simulink model "IIR_filter"  (R2017b)
settings: Solver=VariableStepAuto  StartTime=0.0  StopTime=10.0  RelTol=1e-3
libraries: dspstat3 x4, commutil2 x2, simulink x1
settings Model: Creator=ARNAB KUMAR MONDAL  LastModifiedBy=ARNAB KUMAR MONDAL

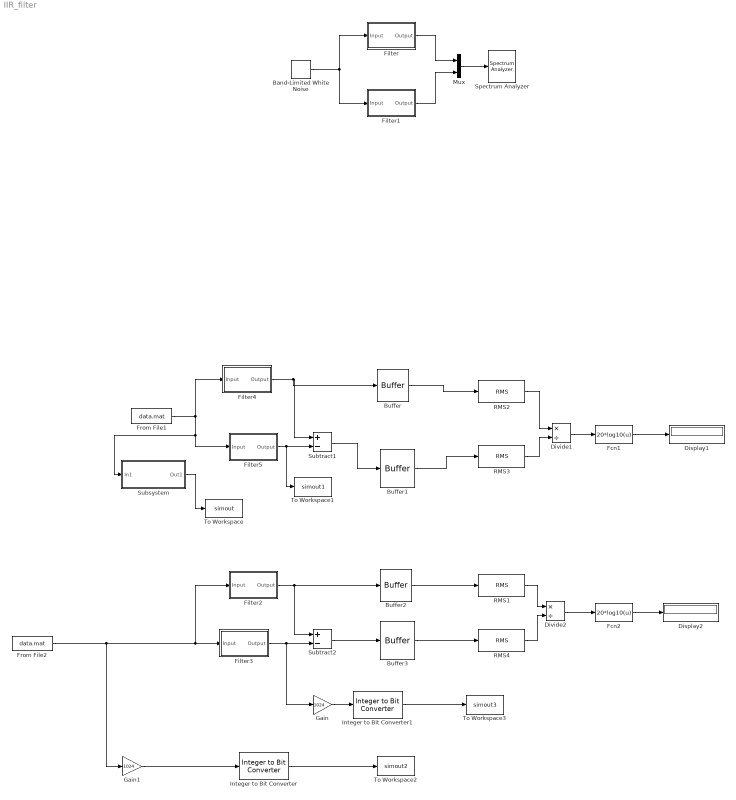
== system IIR_filter ==
  Band-Limited White Noise : simulink/Sources/Band-Limited White Noise  Cov=[1]  Ts=1/44100  seed=[23341]
  Buffer{,1..3} (4 alike) : Buffer  OutputFrames=off
  Display1 : Display
  Display2 : Display
  Divide1 : Product  Inputs=*/
  Divide2 : Product  Inputs=*/
  Fcn1 : Fcn  Expr=20*log10(u)
  Fcn2 : Fcn  Expr=20*log10(u)
  Filter : Subsystem  Tag=FilterWizardSubSystem
      settings: ErrorFcn=dspFilterRealizedInBasicElemsAlgLoopErrFcnCallback
  Filter1 : Subsystem  Tag=FilterWizardSubSystem  mask{k=11, s=4, ck=11}
      settings: ErrorFcn=dspFilterRealizedInBasicElemsAlgLoopErrFcnCallback
  Filter2 : Subsystem  Tag=FilterWizardSubSystem
      settings: ErrorFcn=dspFilterRealizedInBasicElemsAlgLoopErrFcnCallback
  Filter3 : Subsystem  Tag=FilterWizardSubSystem  mask{k=11, s=5, ck=11}
      settings: ErrorFcn=dspFilterRealizedInBasicElemsAlgLoopErrFcnCallback
  Filter4 : Subsystem  Tag=FilterWizardSubSystem
      settings: ErrorFcn=dspFilterRealizedInBasicElemsAlgLoopErrFcnCallback
  Filter5 : Subsystem  Tag=FilterWizardSubSystem  mask{k=8, s=4, ck=11}
      settings: ErrorFcn=dspFilterRealizedInBasicElemsAlgLoopErrFcnCallback
  From File1 : FromFile  FileName=data.mat  SampleTime=1/44100
  From File2 : FromFile  FileName=data.mat  SampleTime=1/44100
  Gain : Gain  Gain=1024
  Gain1 : Gain  Gain=1024
  Integer to Bit Converter : commutil2/Integer to Bit Converter  nbits=32  signedInputValues=Signed  bitOrder=MSB first  outDtype=Same as input
  Integer to Bit Converter1 : commutil2/Integer to Bit Converter  nbits=32  signedInputValues=Signed  bitOrder=MSB first  outDtype=Same as input
  Mux : Mux  Inputs=2
  RMS{1..4} (4 alike) : dspstat3/RMS  run=on  directionMode=Each column  dimension=1  reset_popup=None
  Spectrum Analyzer : SpectrumAnalyzer
  Subsystem : Subsystem  mask{k=8, s=4}
  Subtract1 : Sum  Inputs=+-
  Subtract2 : Sum  Inputs=+-
  To Workspace : ToWorkspace  VariableName=simout  SaveFormat=Timeseries  SampleTime=-1
  To Workspace1 : ToWorkspace  VariableName=simout1  SaveFormat=Timeseries  SampleTime=-1
  To Workspace2 : ToWorkspace  VariableName=simout2  SaveFormat=Timeseries  SampleTime=-1
      settings: Save2DSignal=2-D array (concatenate along first dimension)
  To Workspace3 : ToWorkspace  VariableName=simout3  SaveFormat=Timeseries  SampleTime=-1
      settings: Save2DSignal=2-D array (concatenate along first dimension)
  wires:
  Band-Limited White Noise/1 -> Filter/1(Input), Filter1/1(Input)
  Filter1/1(Output) -> Mux/2
  RMS2/1 -> Divide1/1
  Filter4/1(Output) -> Buffer/1, Subtract1/1
  Divide1/1 -> Fcn1/1
  From File1/1 -> Subsystem/1(In1), Filter5/1(Input), Filter4/1(Input)
  RMS3/1 -> Divide1/2
  Filter5/1(Output) -> To Workspace1/1, Subtract1/2
  Fcn1/1 -> Display1/1
  Subtract1/1 -> Buffer1/1
  Buffer/1 -> RMS2/1
  Buffer1/1 -> RMS3/1
  Fcn2/1 -> Display2/1
  Buffer3/1 -> RMS4/1
  Divide2/1 -> Fcn2/1
  RMS1/1 -> Divide2/1
  Subtract2/1 -> Buffer3/1
  Filter2/1(Output) -> Subtract2/1, Buffer2/1
  RMS4/1 -> Divide2/2
  Buffer2/1 -> RMS1/1
  Filter3/1(Output) -> Gain/1, Subtract2/2
  From File2/1 -> Filter2/1(Input), Filter3/1(Input), Gain1/1
  Subsystem/1(Out1) -> To Workspace/1
  Integer to Bit Converter/1 -> To Workspace2/1
  Integer to Bit Converter1/1 -> To Workspace3/1
  Gain1/1 -> Integer to Bit Converter/1
  Gain/1 -> Integer to Bit Converter1/1
  Filter/1(Output) -> Mux/1
  Mux/1 -> Spectrum Analyzer/1

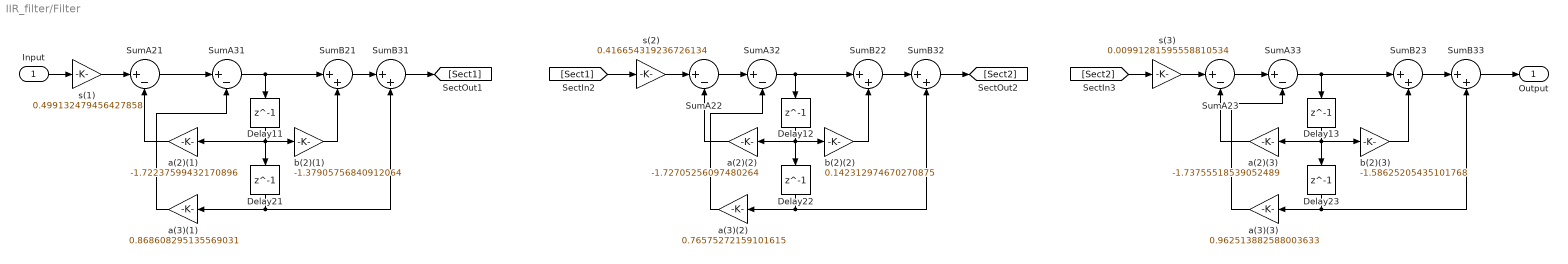
== system IIR_filter/Filter ==
  Input : Inport
  Delay{11..13,21..23} (6 alike) : Delay  DelayLength=1  InitialCondition=0
  SumA{21..23,31..33} (6 alike) : Sum  Inputs=|+-  RndMeth=Nearest  SaturateOnIntegerOverflow=on  OutDataTypeStr=Inherit: Same as first input
  SumB{21..23,31..33} (6 alike) : Sum  Inputs=|++  RndMeth=Nearest  SaturateOnIntegerOverflow=on  OutDataTypeStr=Inherit: Same as first input
  a(2)(1) : Gain  Gain=-1.72237599432170896  ParamDataTypeStr=double  RndMeth=Nearest  SaturateOnIntegerOverflow=on  OutDataTypeStr=Inherit: Same as input
  a(2)(2) : Gain  Gain=-1.72705256097480264  ParamDataTypeStr=double  RndMeth=Nearest  SaturateOnIntegerOverflow=on  OutDataTypeStr=Inherit: Same as input
  a(2)(3) : Gain  Gain=-1.73755518539052489  ParamDataTypeStr=double  RndMeth=Nearest  SaturateOnIntegerOverflow=on  OutDataTypeStr=Inherit: Same as input
  a(3)(1) : Gain  Gain=0.868608295135569031  ParamDataTypeStr=double  RndMeth=Nearest  SaturateOnIntegerOverflow=on  OutDataTypeStr=Inherit: Same as input
  a(3)(2) : Gain  Gain=0.76575272159101615  ParamDataTypeStr=double  RndMeth=Nearest  SaturateOnIntegerOverflow=on  OutDataTypeStr=Inherit: Same as input
  a(3)(3) : Gain  Gain=0.962513882588003633  ParamDataTypeStr=double  RndMeth=Nearest  SaturateOnIntegerOverflow=on  OutDataTypeStr=Inherit: Same as input
  b(2)(1) : Gain  Gain=-1.37905756840912064  ParamDataTypeStr=double  RndMeth=Nearest  SaturateOnIntegerOverflow=on  OutDataTypeStr=Inherit: Same as input
  b(2)(2) : Gain  Gain=0.142312974670270875  ParamDataTypeStr=double  RndMeth=Nearest  SaturateOnIntegerOverflow=on  OutDataTypeStr=Inherit: Same as input
  b(2)(3) : Gain  Gain=-1.58625205435101768  ParamDataTypeStr=double  RndMeth=Nearest  SaturateOnIntegerOverflow=on  OutDataTypeStr=Inherit: Same as input
  s(1) : Gain  Gain=0.499132479456427858  ParamDataTypeStr=double  RndMeth=Nearest  SaturateOnIntegerOverflow=on  OutDataTypeStr=Inherit: Same as input
  s(2) : Gain  Gain=0.416654319236726134  ParamDataTypeStr=double  RndMeth=Nearest  SaturateOnIntegerOverflow=on  OutDataTypeStr=Inherit: Same as input
  s(3) : Gain  Gain=0.00991281595558810534  ParamDataTypeStr=double  RndMeth=Nearest  SaturateOnIntegerOverflow=on  OutDataTypeStr=Inherit: Same as input
  Output : Outport
  wires:
  Input/1 -> s(1)/1
  s(1)/1 -> SumA21/1
  SumA21/1 -> SumA31/1
  SumA31/1 -> SumB21/1, Delay11/1
  SumB21/1 -> SumB31/1
  SumB31/1 -> [Sect1]
  a(2)(1)/1 -> SumA21/2
  Delay11/1 -> b(2)(1)/1, Delay21/1, a(2)(1)/1
  b(2)(1)/1 -> SumB21/2
  a(3)(1)/1 -> SumA31/2
  Delay21/1 -> SumB31/2, a(3)(1)/1
  [Sect1] -> s(2)/1
  s(2)/1 -> SumA22/1
  SumA22/1 -> SumA32/1
  SumA32/1 -> SumB22/1, Delay12/1
  SumB22/1 -> SumB32/1
  SumB32/1 -> [Sect2]
  a(2)(2)/1 -> SumA22/2
  Delay12/1 -> b(2)(2)/1, Delay22/1, a(2)(2)/1
  b(2)(2)/1 -> SumB22/2
  a(3)(2)/1 -> SumA32/2
  Delay22/1 -> SumB32/2, a(3)(2)/1
  b(2)(3)/1 -> SumB23/2
  SumA33/1 -> SumB23/1, Delay13/1
  [Sect2] -> s(3)/1
  Delay23/1 -> SumB33/2, a(3)(3)/1
  Delay13/1 -> b(2)(3)/1, Delay23/1, a(2)(3)/1
  SumB23/1 -> SumB33/1
  SumA23/1 -> SumA33/1
  a(3)(3)/1 -> SumA33/2
  s(3)/1 -> SumA23/1
  a(2)(3)/1 -> SumA23/2
  SumB33/1 -> Output/1

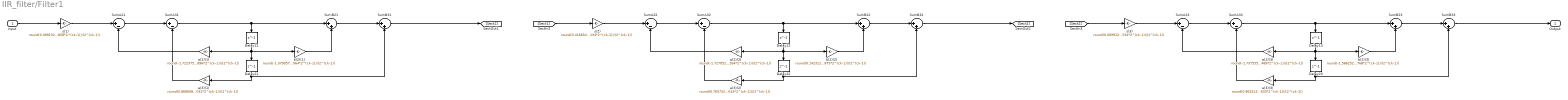
== system IIR_filter/Filter1 ==
  Input : Inport
  Delay{11..13,21..23} (6 alike) : Delay  DelayLength=1  InitialCondition=0
  SumA{21..23,31..33} (6 alike) : Sum  Inputs=|+-  RndMeth=Nearest  SaturateOnIntegerOverflow=on  OutDataTypeStr=Inherit: Same as first input
  SumB{21..23,31..33} (6 alike) : Sum  Inputs=|++  RndMeth=Nearest  SaturateOnIntegerOverflow=on  OutDataTypeStr=Inherit: Same as first input
  a(2)(1) : Gain  Gain=round(-1.72237599432170896*2^(ck-1))/(2^(ck-1))  ParamDataTypeStr=double  RndMeth=Nearest  SaturateOnIntegerOverflow=on  OutDataTypeStr=Inherit: Same as input
  a(2)(2) : Gain  Gain=round(-1.72705256097480264*2^(ck-1))/(2^(ck-1))  ParamDataTypeStr=double  RndMeth=Nearest  SaturateOnIntegerOverflow=on  OutDataTypeStr=Inherit: Same as input
  a(2)(3) : Gain  Gain=round(-1.73755518539052489*2^(ck-1))/(2^(ck-1))  ParamDataTypeStr=double  RndMeth=Nearest  SaturateOnIntegerOverflow=on  OutDataTypeStr=Inherit: Same as input
  a(3)(1) : Gain  Gain=round(0.868608295135569031*2^(ck-1))/(2^(ck-1))  ParamDataTypeStr=double  RndMeth=Nearest  SaturateOnIntegerOverflow=on  OutDataTypeStr=Inherit: Same as input
  a(3)(2) : Gain  Gain=round(0.76575272159101615*2^(ck-1))/(2^(ck-1))  ParamDataTypeStr=double  RndMeth=Nearest  SaturateOnIntegerOverflow=on  OutDataTypeStr=Inherit: Same as input
  a(3)(3) : Gain  Gain=round(0.962513882588003633*2^(ck-1))/(2^(ck-1))  ParamDataTypeStr=double  RndMeth=Nearest  SaturateOnIntegerOverflow=on  OutDataTypeStr=Inherit: Same as input
  b(2)(1) : Gain  Gain=round(-1.37905756840912064*2^(ck-1))/(2^(ck-1))  ParamDataTypeStr=double  RndMeth=Nearest  SaturateOnIntegerOverflow=on  OutDataTypeStr=Inherit: Same as input
  b(2)(2) : Gain  Gain=round(0.142312974670270875*2^(ck-1))/(2^(ck-1))  ParamDataTypeStr=double  RndMeth=Nearest  SaturateOnIntegerOverflow=on  OutDataTypeStr=Inherit: Same as input
  b(2)(3) : Gain  Gain=round(-1.58625205435101768*2^(ck-1))/(2^(ck-1))  ParamDataTypeStr=double  RndMeth=Nearest  SaturateOnIntegerOverflow=on  OutDataTypeStr=Inherit: Same as input
  s(1) : Gain  Gain=round(0.499132479456427858*2^(ck-1))/(2^(ck-1))  ParamDataTypeStr=double  RndMeth=Nearest  SaturateOnIntegerOverflow=on  OutDataTypeStr=Inherit: Same as input
  s(2) : Gain  Gain=round(0.416654319236726134*2^(ck-1))/(2^(ck-1))  ParamDataTypeStr=double  RndMeth=Nearest  SaturateOnIntegerOverflow=on  OutDataTypeStr=Inherit: Same as input
  s(3) : Gain  Gain=round(0.00991281595558810534*2^(ck-1))/(2^(ck-1))  ParamDataTypeStr=double  RndMeth=Nearest  SaturateOnIntegerOverflow=on  OutDataTypeStr=Inherit: Same as input
  Output : Outport
  wires:
  Input/1 -> s(1)/1
  s(1)/1 -> SumA21/1
  SumA21/1 -> SumA31/1
  SumA31/1 -> SumB21/1, Delay11/1
  SumB21/1 -> SumB31/1
  SumB31/1 -> [Sect1]
  a(2)(1)/1 -> SumA21/2
  Delay11/1 -> a(2)(1)/1, b(2)(1)/1, Delay21/1
  b(2)(1)/1 -> SumB21/2
  a(3)(1)/1 -> SumA31/2
  Delay21/1 -> a(3)(1)/1, SumB31/2
  [Sect1] -> s(2)/1
  s(2)/1 -> SumA22/1
  SumA22/1 -> SumA32/1
  SumA32/1 -> SumB22/1, Delay12/1
  SumB22/1 -> SumB32/1
  SumB32/1 -> [Sect2]
  a(2)(2)/1 -> SumA22/2
  Delay12/1 -> a(2)(2)/1, b(2)(2)/1, Delay22/1
  b(2)(2)/1 -> SumB22/2
  a(3)(2)/1 -> SumA32/2
  Delay22/1 -> a(3)(2)/1, SumB32/2
  [Sect2] -> s(3)/1
  s(3)/1 -> SumA23/1
  SumA23/1 -> SumA33/1
  SumA33/1 -> SumB23/1, Delay13/1
  SumB23/1 -> SumB33/1
  SumB33/1 -> Output/1
  a(2)(3)/1 -> SumA23/2
  Delay13/1 -> a(2)(3)/1, b(2)(3)/1, Delay23/1
  b(2)(3)/1 -> SumB23/2
  a(3)(3)/1 -> SumA33/2
  Delay23/1 -> a(3)(3)/1, SumB33/2

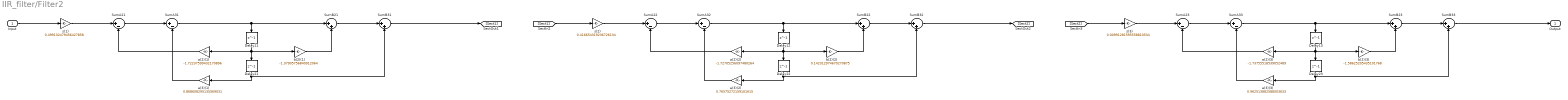
== system IIR_filter/Filter2 ==
  Input : Inport
  Delay{11..13,21..23} (6 alike) : Delay  DelayLength=1  InitialCondition=0
  SumA{21..23,31..33} (6 alike) : Sum  Inputs=|+-  RndMeth=Nearest  SaturateOnIntegerOverflow=on  OutDataTypeStr=Inherit: Same as first input
  SumB{21..23,31..33} (6 alike) : Sum  Inputs=|++  RndMeth=Nearest  SaturateOnIntegerOverflow=on  OutDataTypeStr=Inherit: Same as first input
  a(2)(1) : Gain  Gain=-1.72237599432170896  ParamDataTypeStr=double  RndMeth=Nearest  SaturateOnIntegerOverflow=on  OutDataTypeStr=Inherit: Same as input
  a(2)(2) : Gain  Gain=-1.72705256097480264  ParamDataTypeStr=double  RndMeth=Nearest  SaturateOnIntegerOverflow=on  OutDataTypeStr=Inherit: Same as input
  a(2)(3) : Gain  Gain=-1.73755518539052489  ParamDataTypeStr=double  RndMeth=Nearest  SaturateOnIntegerOverflow=on  OutDataTypeStr=Inherit: Same as input
  a(3)(1) : Gain  Gain=0.868608295135569031  ParamDataTypeStr=double  RndMeth=Nearest  SaturateOnIntegerOverflow=on  OutDataTypeStr=Inherit: Same as input
  a(3)(2) : Gain  Gain=0.76575272159101615  ParamDataTypeStr=double  RndMeth=Nearest  SaturateOnIntegerOverflow=on  OutDataTypeStr=Inherit: Same as input
  a(3)(3) : Gain  Gain=0.962513882588003633  ParamDataTypeStr=double  RndMeth=Nearest  SaturateOnIntegerOverflow=on  OutDataTypeStr=Inherit: Same as input
  b(2)(1) : Gain  Gain=-1.37905756840912064  ParamDataTypeStr=double  RndMeth=Nearest  SaturateOnIntegerOverflow=on  OutDataTypeStr=Inherit: Same as input
  b(2)(2) : Gain  Gain=0.142312974670270875  ParamDataTypeStr=double  RndMeth=Nearest  SaturateOnIntegerOverflow=on  OutDataTypeStr=Inherit: Same as input
  b(2)(3) : Gain  Gain=-1.58625205435101768  ParamDataTypeStr=double  RndMeth=Nearest  SaturateOnIntegerOverflow=on  OutDataTypeStr=Inherit: Same as input
  s(1) : Gain  Gain=0.499132479456427858  ParamDataTypeStr=double  RndMeth=Nearest  SaturateOnIntegerOverflow=on  OutDataTypeStr=Inherit: Same as input
  s(2) : Gain  Gain=0.416654319236726134  ParamDataTypeStr=double  RndMeth=Nearest  SaturateOnIntegerOverflow=on  OutDataTypeStr=Inherit: Same as input
  s(3) : Gain  Gain=0.00991281595558810534  ParamDataTypeStr=double  RndMeth=Nearest  SaturateOnIntegerOverflow=on  OutDataTypeStr=Inherit: Same as input
  Output : Outport
  wires:
  Input/1 -> s(1)/1
  s(1)/1 -> SumA21/1
  SumA21/1 -> SumA31/1
  SumA31/1 -> SumB21/1, Delay11/1
  SumB21/1 -> SumB31/1
  SumB31/1 -> [Sect1]
  a(2)(1)/1 -> SumA21/2
  Delay11/1 -> a(2)(1)/1, b(2)(1)/1, Delay21/1
  b(2)(1)/1 -> SumB21/2
  a(3)(1)/1 -> SumA31/2
  Delay21/1 -> a(3)(1)/1, SumB31/2
  [Sect1] -> s(2)/1
  s(2)/1 -> SumA22/1
  SumA22/1 -> SumA32/1
  SumA32/1 -> SumB22/1, Delay12/1
  SumB22/1 -> SumB32/1
  SumB32/1 -> [Sect2]
  a(2)(2)/1 -> SumA22/2
  Delay12/1 -> a(2)(2)/1, b(2)(2)/1, Delay22/1
  b(2)(2)/1 -> SumB22/2
  a(3)(2)/1 -> SumA32/2
  Delay22/1 -> a(3)(2)/1, SumB32/2
  [Sect2] -> s(3)/1
  s(3)/1 -> SumA23/1
  SumA23/1 -> SumA33/1
  SumA33/1 -> SumB23/1, Delay13/1
  SumB23/1 -> SumB33/1
  SumB33/1 -> Output/1
  a(2)(3)/1 -> SumA23/2
  Delay13/1 -> a(2)(3)/1, b(2)(3)/1, Delay23/1
  b(2)(3)/1 -> SumB23/2
  a(3)(3)/1 -> SumA33/2
  Delay23/1 -> a(3)(3)/1, SumB33/2

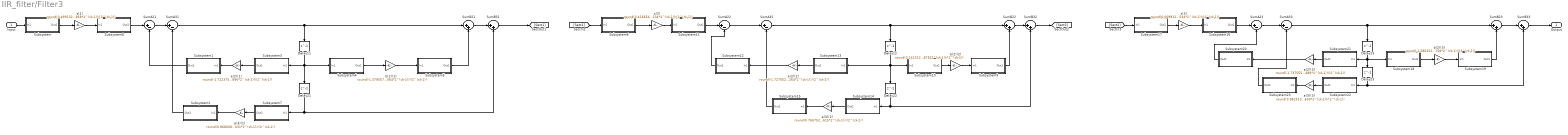
== system IIR_filter/Filter3 ==
  Input : Inport
  Delay{11..13,21..23} (6 alike) : Delay  DelayLength=1  InitialCondition=0
  Subsystem : Subsystem
  Subsystem1 : Subsystem
  Subsystem10 : Subsystem
  Subsystem11 : Subsystem
  Subsystem12 : Subsystem
  Subsystem13 : Subsystem
  Subsystem14 : Subsystem
  Subsystem15 : Subsystem
  Subsystem16 : Subsystem
  Subsystem17 : Subsystem
  Subsystem18 : Subsystem
  Subsystem19 : Subsystem
  Subsystem2 : Subsystem
  Subsystem20 : Subsystem
  Subsystem21 : Subsystem
  Subsystem22 : Subsystem
  Subsystem23 : Subsystem
  Subsystem3 : Subsystem
  Subsystem4 : Subsystem
  Subsystem5 : Subsystem
  Subsystem6 : Subsystem
  Subsystem7 : Subsystem
  Subsystem8 : Subsystem
  Subsystem9 : Subsystem
  SumA{21..23,31..33} (6 alike) : Sum  Inputs=|+-  RndMeth=Nearest  SaturateOnIntegerOverflow=on  OutDataTypeStr=Inherit: Same as first input
  SumB{21..23,31..33} (6 alike) : Sum  Inputs=|++  RndMeth=Nearest  SaturateOnIntegerOverflow=on  OutDataTypeStr=Inherit: Same as first input
  a(2)(1) : Gain  Gain=round(-1.72237599432170896*2^(ck-1))/(2^(ck-1))  ParamDataTypeStr=double  RndMeth=Nearest  SaturateOnIntegerOverflow=on  OutDataTypeStr=Inherit: Same as input
  a(2)(2) : Gain  Gain=round(-1.72705256097480264*2^(ck-1))/(2^(ck-1))  ParamDataTypeStr=double  RndMeth=Nearest  SaturateOnIntegerOverflow=on  OutDataTypeStr=Inherit: Same as input
  a(2)(3) : Gain  Gain=round(-1.73755518539052489*2^(ck-1))/(2^(ck-1))  ParamDataTypeStr=double  RndMeth=Nearest  SaturateOnIntegerOverflow=on  OutDataTypeStr=Inherit: Same as input
  a(3)(1) : Gain  Gain=round(0.868608295135569031*2^(ck-1))/(2^(ck-1))  ParamDataTypeStr=double  RndMeth=Nearest  SaturateOnIntegerOverflow=on  OutDataTypeStr=Inherit: Same as input
  a(3)(2) : Gain  Gain=round(0.76575272159101615*2^(ck-1))/(2^(ck-1))  ParamDataTypeStr=double  RndMeth=Nearest  SaturateOnIntegerOverflow=on  OutDataTypeStr=Inherit: Same as input
  a(3)(3) : Gain  Gain=round(0.962513882588003633*2^(ck-1))/(2^(ck-1))  ParamDataTypeStr=double  RndMeth=Nearest  SaturateOnIntegerOverflow=on  OutDataTypeStr=Inherit: Same as input
  b(2)(1) : Gain  Gain=round(-1.37905756840912064*2^(ck-1))/(2^(ck-1))  ParamDataTypeStr=double  RndMeth=Nearest  SaturateOnIntegerOverflow=on  OutDataTypeStr=Inherit: Same as input
  b(2)(2) : Gain  Gain=round(0.142312974670270875*2^(ck-1))/(2^(ck-1))  ParamDataTypeStr=double  RndMeth=Nearest  SaturateOnIntegerOverflow=on  OutDataTypeStr=Inherit: Same as input
  b(2)(3) : Gain  Gain=round(-1.58625205435101768*2^(ck-1))/(2^(ck-1))  ParamDataTypeStr=double  RndMeth=Nearest  SaturateOnIntegerOverflow=on  OutDataTypeStr=Inherit: Same as input
  s(1) : Gain  Gain=round(0.499132479456427858*2^(ck-1))/(2^(ck-1))  ParamDataTypeStr=double  RndMeth=Nearest  SaturateOnIntegerOverflow=on  OutDataTypeStr=Inherit: Same as input
  s(2) : Gain  Gain=round(0.416654319236726134*2^(ck-1))/(2^(ck-1))  ParamDataTypeStr=double  RndMeth=Nearest  SaturateOnIntegerOverflow=on  OutDataTypeStr=Inherit: Same as input
  s(3) : Gain  Gain=round(0.00991281595558810534*2^(ck-1))/(2^(ck-1))  ParamDataTypeStr=double  RndMeth=Nearest  SaturateOnIntegerOverflow=on  OutDataTypeStr=Inherit: Same as input
  Output : Outport
  wires:
  SumB31/1 -> [Sect1]
  Delay11/1 -> Delay21/1, Subsystem4/1(In1), Subsystem3/1(In1)
  b(2)(1)/1 -> Subsystem5/1(In1)
  a(3)(1)/1 -> Subsystem2/1(In1)
  [Sect1] -> Subsystem6/1(In1)
  s(2)/1 -> Subsystem11/1(In1)
  SumB32/1 -> [Sect2]
  a(2)(2)/1 -> Subsystem12/1(In1)
  Delay12/1 -> Subsystem10/1(In1), Delay22/1, Subsystem13/1(In1)
  b(2)(2)/1 -> Subsystem9/1(In1)
  a(3)(2)/1 -> Subsystem15/1(In1)
  [Sect2] -> Subsystem17/1(In1)
  s(3)/1 -> Subsystem16/1(In1)
  a(2)(3)/1 -> Subsystem20/1(In1)
  Delay13/1 -> Subsystem21/1(In1), Delay23/1, Subsystem18/1(In1)
  b(2)(3)/1 -> Subsystem19/1(In1)
  a(3)(3)/1 -> Subsystem23/1(In1)
  s(1)/1 -> Subsystem8/1(In1)
  a(2)(1)/1 -> Subsystem1/1(In1)
  Input/1 -> Subsystem/1(In1)
  Subsystem/1(Out1) -> s(1)/1
  Subsystem1/1(Out1) -> SumA21/2
  Subsystem2/1(Out1) -> SumA31/2
  Subsystem3/1(Out1) -> a(2)(1)/1
  Subsystem4/1(Out1) -> b(2)(1)/1
  Subsystem5/1(Out1) -> SumB21/2
  Subsystem6/1(Out1) -> s(2)/1
  Subsystem7/1(Out1) -> a(3)(1)/1
  Subsystem8/1(Out1) -> SumA21/1
  Subsystem9/1(Out1) -> SumB22/2
  Subsystem10/1(Out1) -> b(2)(2)/1
  Subsystem11/1(Out1) -> SumA22/1
  Subsystem13/1(Out1) -> a(2)(2)/1
  Subsystem14/1(Out1) -> a(3)(2)/1
  Subsystem12/1(Out1) -> SumA22/2
  Subsystem15/1(Out1) -> SumA32/2
  Subsystem17/1(Out1) -> s(3)/1
  Subsystem19/1(Out1) -> SumB23/2
  Subsystem18/1(Out1) -> b(2)(3)/1
  Subsystem20/1(Out1) -> SumA23/2
  Subsystem21/1(Out1) -> a(2)(3)/1
  Subsystem22/1(Out1) -> a(3)(3)/1
  Subsystem23/1(Out1) -> SumA33/2
  Subsystem16/1(Out1) -> SumA23/1
  Delay21/1 -> SumB31/2, Subsystem7/1(In1)
  Delay22/1 -> SumB32/2, Subsystem14/1(In1)
  Delay23/1 -> SumB33/2, Subsystem22/1(In1)
  SumA21/1 -> SumA31/1
  SumB21/1 -> SumB31/1
  SumA22/1 -> SumA32/1
  SumB22/1 -> SumB32/1
  SumA23/1 -> SumA33/1
  SumB23/1 -> SumB33/1
  SumB33/1 -> Output/1
  SumA33/1 -> SumB23/1, Delay13/1
  SumA32/1 -> SumB22/1, Delay12/1
  SumA31/1 -> SumB21/1, Delay11/1

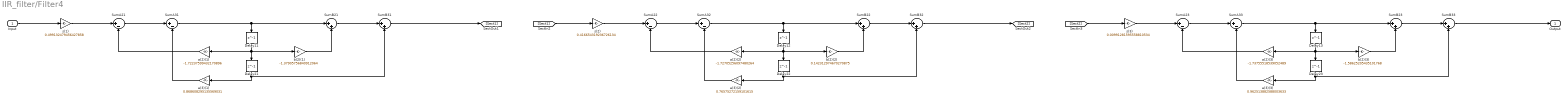
== system IIR_filter/Filter4 ==
  Input : Inport
  Delay{11..13,21..23} (6 alike) : Delay  DelayLength=1  InitialCondition=0
  SumA{21..23,31..33} (6 alike) : Sum  Inputs=|+-  RndMeth=Nearest  SaturateOnIntegerOverflow=on  OutDataTypeStr=Inherit: Same as first input
  SumB{21..23,31..33} (6 alike) : Sum  Inputs=|++  RndMeth=Nearest  SaturateOnIntegerOverflow=on  OutDataTypeStr=Inherit: Same as first input
  a(2)(1) : Gain  Gain=-1.72237599432170896  ParamDataTypeStr=double  RndMeth=Nearest  SaturateOnIntegerOverflow=on  OutDataTypeStr=Inherit: Same as input
  a(2)(2) : Gain  Gain=-1.72705256097480264  ParamDataTypeStr=double  RndMeth=Nearest  SaturateOnIntegerOverflow=on  OutDataTypeStr=Inherit: Same as input
  a(2)(3) : Gain  Gain=-1.73755518539052489  ParamDataTypeStr=double  RndMeth=Nearest  SaturateOnIntegerOverflow=on  OutDataTypeStr=Inherit: Same as input
  a(3)(1) : Gain  Gain=0.868608295135569031  ParamDataTypeStr=double  RndMeth=Nearest  SaturateOnIntegerOverflow=on  OutDataTypeStr=Inherit: Same as input
  a(3)(2) : Gain  Gain=0.76575272159101615  ParamDataTypeStr=double  RndMeth=Nearest  SaturateOnIntegerOverflow=on  OutDataTypeStr=Inherit: Same as input
  a(3)(3) : Gain  Gain=0.962513882588003633  ParamDataTypeStr=double  RndMeth=Nearest  SaturateOnIntegerOverflow=on  OutDataTypeStr=Inherit: Same as input
  b(2)(1) : Gain  Gain=-1.37905756840912064  ParamDataTypeStr=double  RndMeth=Nearest  SaturateOnIntegerOverflow=on  OutDataTypeStr=Inherit: Same as input
  b(2)(2) : Gain  Gain=0.142312974670270875  ParamDataTypeStr=double  RndMeth=Nearest  SaturateOnIntegerOverflow=on  OutDataTypeStr=Inherit: Same as input
  b(2)(3) : Gain  Gain=-1.58625205435101768  ParamDataTypeStr=double  RndMeth=Nearest  SaturateOnIntegerOverflow=on  OutDataTypeStr=Inherit: Same as input
  s(1) : Gain  Gain=0.499132479456427858  ParamDataTypeStr=double  RndMeth=Nearest  SaturateOnIntegerOverflow=on  OutDataTypeStr=Inherit: Same as input
  s(2) : Gain  Gain=0.416654319236726134  ParamDataTypeStr=double  RndMeth=Nearest  SaturateOnIntegerOverflow=on  OutDataTypeStr=Inherit: Same as input
  s(3) : Gain  Gain=0.00991281595558810534  ParamDataTypeStr=double  RndMeth=Nearest  SaturateOnIntegerOverflow=on  OutDataTypeStr=Inherit: Same as input
  Output : Outport
  wires:
  Input/1 -> s(1)/1
  s(1)/1 -> SumA21/1
  SumA21/1 -> SumA31/1
  SumA31/1 -> SumB21/1, Delay11/1
  SumB21/1 -> SumB31/1
  SumB31/1 -> [Sect1]
  a(2)(1)/1 -> SumA21/2
  Delay11/1 -> a(2)(1)/1, b(2)(1)/1, Delay21/1
  b(2)(1)/1 -> SumB21/2
  a(3)(1)/1 -> SumA31/2
  Delay21/1 -> a(3)(1)/1, SumB31/2
  [Sect1] -> s(2)/1
  s(2)/1 -> SumA22/1
  SumA22/1 -> SumA32/1
  SumA32/1 -> SumB22/1, Delay12/1
  SumB22/1 -> SumB32/1
  SumB32/1 -> [Sect2]
  a(2)(2)/1 -> SumA22/2
  Delay12/1 -> a(2)(2)/1, b(2)(2)/1, Delay22/1
  b(2)(2)/1 -> SumB22/2
  a(3)(2)/1 -> SumA32/2
  Delay22/1 -> a(3)(2)/1, SumB32/2
  [Sect2] -> s(3)/1
  s(3)/1 -> SumA23/1
  SumA23/1 -> SumA33/1
  SumA33/1 -> SumB23/1, Delay13/1
  SumB23/1 -> SumB33/1
  SumB33/1 -> Output/1
  a(2)(3)/1 -> SumA23/2
  Delay13/1 -> a(2)(3)/1, b(2)(3)/1, Delay23/1
  b(2)(3)/1 -> SumB23/2
  a(3)(3)/1 -> SumA33/2
  Delay23/1 -> a(3)(3)/1, SumB33/2

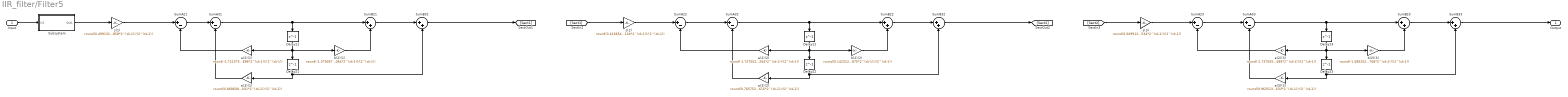
== system IIR_filter/Filter5 ==
  Input : Inport
  Delay{11..13,21..23} (6 alike) : Delay  DelayLength=1  InitialCondition=0
  Subsystem : Subsystem
  SumA{21..23,31..33} (6 alike) : Sum  Inputs=|+-  RndMeth=Nearest  SaturateOnIntegerOverflow=on  OutDataTypeStr=Inherit: Same as first input
  SumB{21..23,31..33} (6 alike) : Sum  Inputs=|++  RndMeth=Nearest  SaturateOnIntegerOverflow=on  OutDataTypeStr=Inherit: Same as first input
  a(2)(1) : Gain  Gain=round(-1.72237599432170896*2^(ck-1))/(2^(ck-1))  ParamDataTypeStr=double  RndMeth=Nearest  SaturateOnIntegerOverflow=on  OutDataTypeStr=Inherit: Same as input
  a(2)(2) : Gain  Gain=round(-1.72705256097480264*2^(ck-1))/(2^(ck-1))  ParamDataTypeStr=double  RndMeth=Nearest  SaturateOnIntegerOverflow=on  OutDataTypeStr=Inherit: Same as input
  a(2)(3) : Gain  Gain=round(-1.73755518539052489*2^(ck-1))/(2^(ck-1))  ParamDataTypeStr=double  RndMeth=Nearest  SaturateOnIntegerOverflow=on  OutDataTypeStr=Inherit: Same as input
  a(3)(1) : Gain  Gain=round(0.868608295135569031*2^(ck-1))/(2^(ck-1))  ParamDataTypeStr=double  RndMeth=Nearest  SaturateOnIntegerOverflow=on  OutDataTypeStr=Inherit: Same as input
  a(3)(2) : Gain  Gain=round(0.76575272159101615*2^(ck-1))/(2^(ck-1))  ParamDataTypeStr=double  RndMeth=Nearest  SaturateOnIntegerOverflow=on  OutDataTypeStr=Inherit: Same as input
  a(3)(3) : Gain  Gain=round(0.962513882588003633*2^(ck-1))/(2^(ck-1))  ParamDataTypeStr=double  RndMeth=Nearest  SaturateOnIntegerOverflow=on  OutDataTypeStr=Inherit: Same as input
  b(2)(1) : Gain  Gain=round(-1.37905756840912064*2^(ck-1))/(2^(ck-1))  ParamDataTypeStr=double  RndMeth=Nearest  SaturateOnIntegerOverflow=on  OutDataTypeStr=Inherit: Same as input
  b(2)(2) : Gain  Gain=round(0.142312974670270875*2^(ck-1))/(2^(ck-1))  ParamDataTypeStr=double  RndMeth=Nearest  SaturateOnIntegerOverflow=on  OutDataTypeStr=Inherit: Same as input
  b(2)(3) : Gain  Gain=round(-1.58625205435101768*2^(ck-1))/(2^(ck-1))  ParamDataTypeStr=double  RndMeth=Nearest  SaturateOnIntegerOverflow=on  OutDataTypeStr=Inherit: Same as input
  s(1) : Gain  Gain=round(0.499132479456427858*2^(ck-1))/(2^(ck-1))  ParamDataTypeStr=double  RndMeth=Nearest  SaturateOnIntegerOverflow=on  OutDataTypeStr=Inherit: Same as input
  s(2) : Gain  Gain=round(0.416654319236726134*2^(ck-1))/(2^(ck-1))  ParamDataTypeStr=double  RndMeth=Nearest  SaturateOnIntegerOverflow=on  OutDataTypeStr=Inherit: Same as input
  s(3) : Gain  Gain=round(0.00991281595558810534*2^(ck-1))/(2^(ck-1))  ParamDataTypeStr=double  RndMeth=Nearest  SaturateOnIntegerOverflow=on  OutDataTypeStr=Inherit: Same as input
  Output : Outport
  wires:
  SumB21/1 -> SumB31/1
  SumB31/1 -> [Sect1]
  Delay11/1 -> a(2)(1)/1, b(2)(1)/1, Delay21/1
  b(2)(1)/1 -> SumB21/2
  a(3)(1)/1 -> SumA31/2
  Delay21/1 -> a(3)(1)/1, SumB31/2
  [Sect1] -> s(2)/1
  s(2)/1 -> SumA22/1
  SumA22/1 -> SumA32/1
  SumA32/1 -> SumB22/1, Delay12/1
  SumB22/1 -> SumB32/1
  SumB32/1 -> [Sect2]
  a(2)(2)/1 -> SumA22/2
  Delay12/1 -> a(2)(2)/1, b(2)(2)/1, Delay22/1
  b(2)(2)/1 -> SumB22/2
  a(3)(2)/1 -> SumA32/2
  Delay22/1 -> a(3)(2)/1, SumB32/2
  [Sect2] -> s(3)/1
  s(3)/1 -> SumA23/1
  SumA23/1 -> SumA33/1
  SumA33/1 -> SumB23/1, Delay13/1
  SumB23/1 -> SumB33/1
  a(2)(3)/1 -> SumA23/2
  Delay13/1 -> a(2)(3)/1, b(2)(3)/1, Delay23/1
  b(2)(3)/1 -> SumB23/2
  a(3)(3)/1 -> SumA33/2
  Delay23/1 -> a(3)(3)/1, SumB33/2
  s(1)/1 -> SumA21/1
  SumA21/1 -> SumA31/1
  a(2)(1)/1 -> SumA21/2
  SumA31/1 -> SumB21/1, Delay11/1
  Input/1 -> Subsystem/1(In1)
  Subsystem/1(Out1) -> s(1)/1
  SumB33/1 -> Output/1

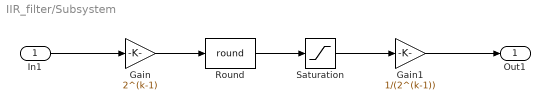
== system IIR_filter/Subsystem ==
  In1 : Inport
  Gain : Gain  Gain=2^(k-1)
  Gain1 : Gain  Gain=1/(2^(k-1))
  Round : Rounding  Operator=round
  Saturation : Saturate  UpperLimit=2^(k+s+-1)-1  LowerLimit=-2^(k+s-1)
  Out1 : Outport
  wires:
  Round/1 -> Saturation/1
  Saturation/1 -> Gain1/1
  Gain/1 -> Round/1
  In1/1 -> Gain/1
  Gain1/1 -> Out1/1

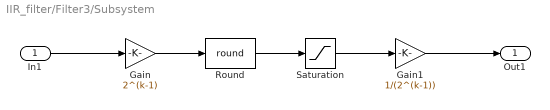
== system IIR_filter/Filter3/Subsystem ==
  In1 : Inport
  Gain : Gain  Gain=2^(k-1)
  Gain1 : Gain  Gain=1/(2^(k-1))
  Round : Rounding  Operator=round
  Saturation : Saturate  UpperLimit=2^(k+s+-1)-1  LowerLimit=-2^(k+s-1)
  Out1 : Outport
  wires:
  Round/1 -> Saturation/1
  Saturation/1 -> Gain1/1
  Gain/1 -> Round/1
  In1/1 -> Gain/1
  Gain1/1 -> Out1/1

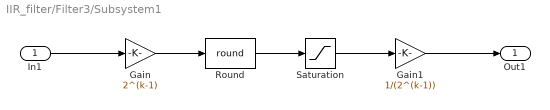
== system IIR_filter/Filter3/Subsystem1 ==
  In1 : Inport
  Gain : Gain  Gain=2^(k-1)
  Gain1 : Gain  Gain=1/(2^(k-1))
  Round : Rounding  Operator=round
  Saturation : Saturate  UpperLimit=2^(k+s+-1)-1  LowerLimit=-2^(k+s-1)
  Out1 : Outport
  wires:
  Round/1 -> Saturation/1
  Saturation/1 -> Gain1/1
  Gain/1 -> Round/1
  In1/1 -> Gain/1
  Gain1/1 -> Out1/1

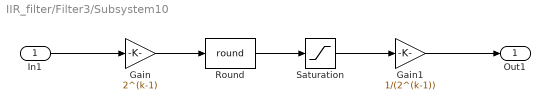
== system IIR_filter/Filter3/Subsystem10 ==
  In1 : Inport
  Gain : Gain  Gain=2^(k-1)
  Gain1 : Gain  Gain=1/(2^(k-1))
  Round : Rounding  Operator=round
  Saturation : Saturate  UpperLimit=2^(k+s+-1)-1  LowerLimit=-2^(k+s-1)
  Out1 : Outport
  wires:
  Round/1 -> Saturation/1
  Saturation/1 -> Gain1/1
  Gain/1 -> Round/1
  In1/1 -> Gain/1
  Gain1/1 -> Out1/1

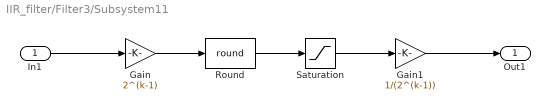
== system IIR_filter/Filter3/Subsystem11 ==
  In1 : Inport
  Gain : Gain  Gain=2^(k-1)
  Gain1 : Gain  Gain=1/(2^(k-1))
  Round : Rounding  Operator=round
  Saturation : Saturate  UpperLimit=2^(k+s+-1)-1  LowerLimit=-2^(k+s-1)
  Out1 : Outport
  wires:
  Round/1 -> Saturation/1
  Saturation/1 -> Gain1/1
  Gain/1 -> Round/1
  In1/1 -> Gain/1
  Gain1/1 -> Out1/1

== system IIR_filter/Filter3/Subsystem12 ==
  In1 : Inport
  Gain : Gain  Gain=2^(k-1)
  Gain1 : Gain  Gain=1/(2^(k-1))
  Round : Rounding  Operator=round
  Saturation : Saturate  UpperLimit=2^(k+s+-1)-1  LowerLimit=-2^(k+s-1)
  Out1 : Outport
  wires:
  Round/1 -> Saturation/1
  Saturation/1 -> Gain1/1
  Gain/1 -> Round/1
  In1/1 -> Gain/1
  Gain1/1 -> Out1/1

== system IIR_filter/Filter3/Subsystem13 ==
  In1 : Inport
  Gain : Gain  Gain=2^(k-1)
  Gain1 : Gain  Gain=1/(2^(k-1))
  Round : Rounding  Operator=round
  Saturation : Saturate  UpperLimit=2^(k+s+-1)-1  LowerLimit=-2^(k+s-1)
  Out1 : Outport
  wires:
  Round/1 -> Saturation/1
  Saturation/1 -> Gain1/1
  Gain/1 -> Round/1
  In1/1 -> Gain/1
  Gain1/1 -> Out1/1

== system IIR_filter/Filter3/Subsystem14 ==
  In1 : Inport
  Gain : Gain  Gain=2^(k-1)
  Gain1 : Gain  Gain=1/(2^(k-1))
  Round : Rounding  Operator=round
  Saturation : Saturate  UpperLimit=2^(k+s+-1)-1  LowerLimit=-2^(k+s-1)
  Out1 : Outport
  wires:
  Round/1 -> Saturation/1
  Saturation/1 -> Gain1/1
  Gain/1 -> Round/1
  In1/1 -> Gain/1
  Gain1/1 -> Out1/1

== system IIR_filter/Filter3/Subsystem15 ==
  In1 : Inport
  Gain : Gain  Gain=2^(k-1)
  Gain1 : Gain  Gain=1/(2^(k-1))
  Round : Rounding  Operator=round
  Saturation : Saturate  UpperLimit=2^(k+s+-1)-1  LowerLimit=-2^(k+s-1)
  Out1 : Outport
  wires:
  Round/1 -> Saturation/1
  Saturation/1 -> Gain1/1
  Gain/1 -> Round/1
  In1/1 -> Gain/1
  Gain1/1 -> Out1/1

== system IIR_filter/Filter3/Subsystem16 ==
  In1 : Inport
  Gain : Gain  Gain=2^(k-1)
  Gain1 : Gain  Gain=1/(2^(k-1))
  Round : Rounding  Operator=round
  Saturation : Saturate  UpperLimit=2^(k+s+-1)-1  LowerLimit=-2^(k+s-1)
  Out1 : Outport
  wires:
  Round/1 -> Saturation/1
  Saturation/1 -> Gain1/1
  Gain/1 -> Round/1
  In1/1 -> Gain/1
  Gain1/1 -> Out1/1

== system IIR_filter/Filter3/Subsystem17 ==
  In1 : Inport
  Gain : Gain  Gain=2^(k-1)
  Gain1 : Gain  Gain=1/(2^(k-1))
  Round : Rounding  Operator=round
  Saturation : Saturate  UpperLimit=2^(k+s+-1)-1  LowerLimit=-2^(k+s-1)
  Out1 : Outport
  wires:
  Round/1 -> Saturation/1
  Saturation/1 -> Gain1/1
  Gain/1 -> Round/1
  In1/1 -> Gain/1
  Gain1/1 -> Out1/1

== system IIR_filter/Filter3/Subsystem18 ==
  In1 : Inport
  Gain : Gain  Gain=2^(k-1)
  Gain1 : Gain  Gain=1/(2^(k-1))
  Round : Rounding  Operator=round
  Saturation : Saturate  UpperLimit=2^(k+s+-1)-1  LowerLimit=-2^(k+s-1)
  Out1 : Outport
  wires:
  Round/1 -> Saturation/1
  Saturation/1 -> Gain1/1
  Gain/1 -> Round/1
  In1/1 -> Gain/1
  Gain1/1 -> Out1/1

== system IIR_filter/Filter3/Subsystem19 ==
  In1 : Inport
  Gain : Gain  Gain=2^(k-1)
  Gain1 : Gain  Gain=1/(2^(k-1))
  Round : Rounding  Operator=round
  Saturation : Saturate  UpperLimit=2^(k+s+-1)-1  LowerLimit=-2^(k+s-1)
  Out1 : Outport
  wires:
  Round/1 -> Saturation/1
  Saturation/1 -> Gain1/1
  Gain/1 -> Round/1
  In1/1 -> Gain/1
  Gain1/1 -> Out1/1

== system IIR_filter/Filter3/Subsystem2 ==
  In1 : Inport
  Gain : Gain  Gain=2^(k-1)
  Gain1 : Gain  Gain=1/(2^(k-1))
  Round : Rounding  Operator=round
  Saturation : Saturate  UpperLimit=2^(k+s+-1)-1  LowerLimit=-2^(k+s-1)
  Out1 : Outport
  wires:
  Round/1 -> Saturation/1
  Saturation/1 -> Gain1/1
  Gain/1 -> Round/1
  In1/1 -> Gain/1
  Gain1/1 -> Out1/1

== system IIR_filter/Filter3/Subsystem20 ==
  In1 : Inport
  Gain : Gain  Gain=2^(k-1)
  Gain1 : Gain  Gain=1/(2^(k-1))
  Round : Rounding  Operator=round
  Saturation : Saturate  UpperLimit=2^(k+s+-1)-1  LowerLimit=-2^(k+s-1)
  Out1 : Outport
  wires:
  Round/1 -> Saturation/1
  Saturation/1 -> Gain1/1
  Gain/1 -> Round/1
  In1/1 -> Gain/1
  Gain1/1 -> Out1/1

== system IIR_filter/Filter3/Subsystem21 ==
  In1 : Inport
  Gain : Gain  Gain=2^(k-1)
  Gain1 : Gain  Gain=1/(2^(k-1))
  Round : Rounding  Operator=round
  Saturation : Saturate  UpperLimit=2^(k+s+-1)-1  LowerLimit=-2^(k+s-1)
  Out1 : Outport
  wires:
  Round/1 -> Saturation/1
  Saturation/1 -> Gain1/1
  Gain/1 -> Round/1
  In1/1 -> Gain/1
  Gain1/1 -> Out1/1

== system IIR_filter/Filter3/Subsystem22 ==
  In1 : Inport
  Gain : Gain  Gain=2^(k-1)
  Gain1 : Gain  Gain=1/(2^(k-1))
  Round : Rounding  Operator=round
  Saturation : Saturate  UpperLimit=2^(k+s+-1)-1  LowerLimit=-2^(k+s-1)
  Out1 : Outport
  wires:
  Round/1 -> Saturation/1
  Saturation/1 -> Gain1/1
  Gain/1 -> Round/1
  In1/1 -> Gain/1
  Gain1/1 -> Out1/1

== system IIR_filter/Filter3/Subsystem23 ==
  In1 : Inport
  Gain : Gain  Gain=2^(k-1)
  Gain1 : Gain  Gain=1/(2^(k-1))
  Round : Rounding  Operator=round
  Saturation : Saturate  UpperLimit=2^(k+s+-1)-1  LowerLimit=-2^(k+s-1)
  Out1 : Outport
  wires:
  Round/1 -> Saturation/1
  Saturation/1 -> Gain1/1
  Gain/1 -> Round/1
  In1/1 -> Gain/1
  Gain1/1 -> Out1/1

== system IIR_filter/Filter3/Subsystem3 ==
  In1 : Inport
  Gain : Gain  Gain=2^(k-1)
  Gain1 : Gain  Gain=1/(2^(k-1))
  Round : Rounding  Operator=round
  Saturation : Saturate  UpperLimit=2^(k+s+-1)-1  LowerLimit=-2^(k+s-1)
  Out1 : Outport
  wires:
  Round/1 -> Saturation/1
  Saturation/1 -> Gain1/1
  Gain/1 -> Round/1
  In1/1 -> Gain/1
  Gain1/1 -> Out1/1

== system IIR_filter/Filter3/Subsystem4 ==
  In1 : Inport
  Gain : Gain  Gain=2^(k-1)
  Gain1 : Gain  Gain=1/(2^(k-1))
  Round : Rounding  Operator=round
  Saturation : Saturate  UpperLimit=2^(k+s+-1)-1  LowerLimit=-2^(k+s-1)
  Out1 : Outport
  wires:
  Round/1 -> Saturation/1
  Saturation/1 -> Gain1/1
  Gain/1 -> Round/1
  In1/1 -> Gain/1
  Gain1/1 -> Out1/1

== system IIR_filter/Filter3/Subsystem5 ==
  In1 : Inport
  Gain : Gain  Gain=2^(k-1)
  Gain1 : Gain  Gain=1/(2^(k-1))
  Round : Rounding  Operator=round
  Saturation : Saturate  UpperLimit=2^(k+s+-1)-1  LowerLimit=-2^(k+s-1)
  Out1 : Outport
  wires:
  Round/1 -> Saturation/1
  Saturation/1 -> Gain1/1
  Gain/1 -> Round/1
  In1/1 -> Gain/1
  Gain1/1 -> Out1/1

== system IIR_filter/Filter3/Subsystem6 ==
  In1 : Inport
  Gain : Gain  Gain=2^(k-1)
  Gain1 : Gain  Gain=1/(2^(k-1))
  Round : Rounding  Operator=round
  Saturation : Saturate  UpperLimit=2^(k+s+-1)-1  LowerLimit=-2^(k+s-1)
  Out1 : Outport
  wires:
  Round/1 -> Saturation/1
  Saturation/1 -> Gain1/1
  Gain/1 -> Round/1
  In1/1 -> Gain/1
  Gain1/1 -> Out1/1

== system IIR_filter/Filter3/Subsystem7 ==
  In1 : Inport
  Gain : Gain  Gain=2^(k-1)
  Gain1 : Gain  Gain=1/(2^(k-1))
  Round : Rounding  Operator=round
  Saturation : Saturate  UpperLimit=2^(k+s+-1)-1  LowerLimit=-2^(k+s-1)
  Out1 : Outport
  wires:
  Round/1 -> Saturation/1
  Saturation/1 -> Gain1/1
  Gain/1 -> Round/1
  In1/1 -> Gain/1
  Gain1/1 -> Out1/1

== system IIR_filter/Filter3/Subsystem8 ==
  In1 : Inport
  Gain : Gain  Gain=2^(k-1)
  Gain1 : Gain  Gain=1/(2^(k-1))
  Round : Rounding  Operator=round
  Saturation : Saturate  UpperLimit=2^(k+s+-1)-1  LowerLimit=-2^(k+s-1)
  Out1 : Outport
  wires:
  Round/1 -> Saturation/1
  Saturation/1 -> Gain1/1
  Gain/1 -> Round/1
  In1/1 -> Gain/1
  Gain1/1 -> Out1/1

== system IIR_filter/Filter3/Subsystem9 ==
  In1 : Inport
  Gain : Gain  Gain=2^(k-1)
  Gain1 : Gain  Gain=1/(2^(k-1))
  Round : Rounding  Operator=round
  Saturation : Saturate  UpperLimit=2^(k+s+-1)-1  LowerLimit=-2^(k+s-1)
  Out1 : Outport
  wires:
  Round/1 -> Saturation/1
  Saturation/1 -> Gain1/1
  Gain/1 -> Round/1
  In1/1 -> Gain/1
  Gain1/1 -> Out1/1

== system IIR_filter/Filter5/Subsystem ==
  In1 : Inport
  Gain : Gain  Gain=2^(k-1)
  Gain1 : Gain  Gain=1/(2^(k-1))
  Round : Rounding  Operator=round
  Saturation : Saturate  UpperLimit=2^(k+s+-1)-1  LowerLimit=-2^(k+s-1)
  Out1 : Outport
  wires:
  Round/1 -> Saturation/1
  Saturation/1 -> Gain1/1
  Gain/1 -> Round/1
  In1/1 -> Gain/1
  Gain1/1 -> Out1/1
